simulink model "Pendulolinealizacion"  (R2022b)
settings: Solver=VariableStepAuto  StartTime=0.0  StopTime=100  FixedStep=0.01  MaxStep=0.1  MinStep=0.01  RelTol=1e-3
model workspace (MAT data in the model file):
  K = 0.3
  W = 1.25
  k = 0.3
  w = 1.25
  x0 = 0
  y0 = 0
undefined symbols (not defined in the file): A, B, C, D, vec
settings Model: NumberOfSteps=10  Creator=WINDOWS  LastModifiedBy=WINDOWS
settings DataIOCC: SaveFormat=Array  OutputTimes=tout

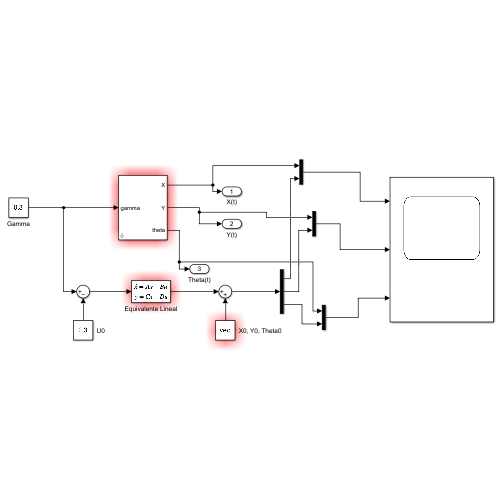
[thumbnail: Simulink's stored preview of the top-level diagram]
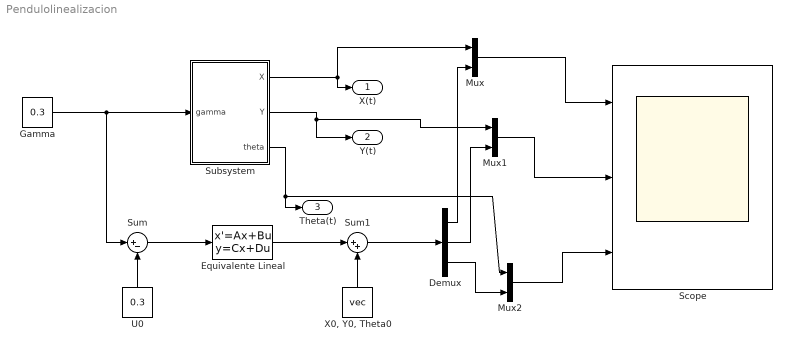
== system Pendulolinealizacion ==
  Demux : Demux  Outputs=3
  Equivalente Lineal : StateSpace  A=A  B=B  C=C  D=D  InitialCondition=0
  Gamma : Constant  Value=0.3
  Mux : Mux  Inputs=2
  Mux1 : Mux  Inputs=2
  Mux2 : Mux  Inputs=2
  Scope : Scope  NumInputPorts=3
  Subsystem : Subsystem  mask{k=k, w=w, x0=vec(1), y0=vec(2), theta0=vec(3)}
  Sum : Sum  Inputs=|+-
  Sum1 : Sum  Inputs=|++
  U0 : Constant  Value=0.3
  "X0, Y0, Theta0" : Constant  Value=vec
  X(t) : Outport
  Y(t) : Outport  Port=2
  Theta(t) : Outport  Port=3
  wires:
  Gamma/1 -> Sum/1, Subsystem/1(gamma)
  Subsystem/1(X) -> X(t)/1, Mux/1
  Subsystem/2(Y) -> Y(t)/1, Mux1/1
  Sum/1 -> Equivalente Lineal/1
  U0/1 -> Sum/2
  Equivalente Lineal/1 -> Sum1/1
  "X0, Y0, Theta0"/1 -> Sum1/2
  Sum1/1 -> Demux/1
  Demux/1 -> Mux/2
  Mux/1 -> Scope/1
  Mux1/1 -> Scope/2
  Demux/2 -> Mux1/2
  Subsystem/3(theta) -> Theta(t)/1, Mux2/1
  Demux/3 -> Mux2/2
  Mux2/1 -> Scope/3

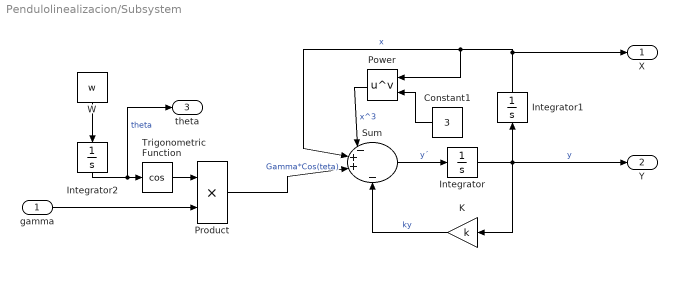
== system Pendulolinealizacion/Subsystem ==
  gamma : Inport
  Constant1 : Constant  Value=3
  Integrator : Integrator  InitialCondition=y0
  Integrator1 : Integrator  InitialCondition=x0
  Integrator2 : Integrator  InitialCondition=theta0
  K : Gain  Gain=k
  Power : Math  Operator=pow
  Product : Product
  Sum : Sum  Inputs=|-++|-
  Trigonometric Function : Trigonometry  Operator=cos
  W : Constant  Value=w
  X : Outport
  Y : Outport  Port=2
  theta : Outport  Port=3
  wires:
  Trigonometric Function/1 -> Product/1
  Integrator/1 -> Y/1, K/1, Integrator1/1  "y"
  Product/1 -> Sum/3  "Gamma*Cos(teta)"
  Power/1 -> Sum/1  "x^3"
  Constant1/1 -> Power/2
  K/1 -> Sum/4  "ky"
  Integrator1/1 -> Power/1, Sum/2, X/1  "x"
  gamma/1 -> Product/2
  Sum/1 -> Integrator/1  "y´"
  Integrator2/1 -> theta/1, Trigonometric Function/1  "theta"
  W/1 -> Integrator2/1
